simulink model "MMNNsExample1"  (R2014a)
settings: Solver=ode45  StartTime=0.0  StopTime=5  RelTol=1e-6
(part 2 of 2)

== system MMNNsExample1/b22(2)(x2(t))*f(x2(t-tau2(t)))/x2(t)*b22(x2(t)) ==
  In1 : Inport
  In2 : Inport  Port=2
  Product1 : Product  RndMeth=Zero
  Variable Time Delay : VariableTransportDelay  MaximumDelay=10  MaximumPoints=2^20
  f(x(t))=0.5*(|x+1|-|x-1|) : Subsystem
  tau2(t)=0.5+0.5*sin(t) : Subsystem
  Out1 : Outport
  wires:
  Product1/1 -> Out1/1
  f(x(t))=0.5*(|x+1|-|x-1|)/1(Out1) -> Variable Time Delay/1
  Variable Time Delay/1 -> Product1/2  "f2(x2(t-tau2(t)))"
  tau2(t)=0.5+0.5*sin(t)/1(Out1) -> Variable Time Delay/2
  In2/1 -> f(x(t))=0.5*(|x+1|-|x-1|)/1(In1)  "x2(t)"
  In1/1 -> Product1/1  "b22(x2(t))"

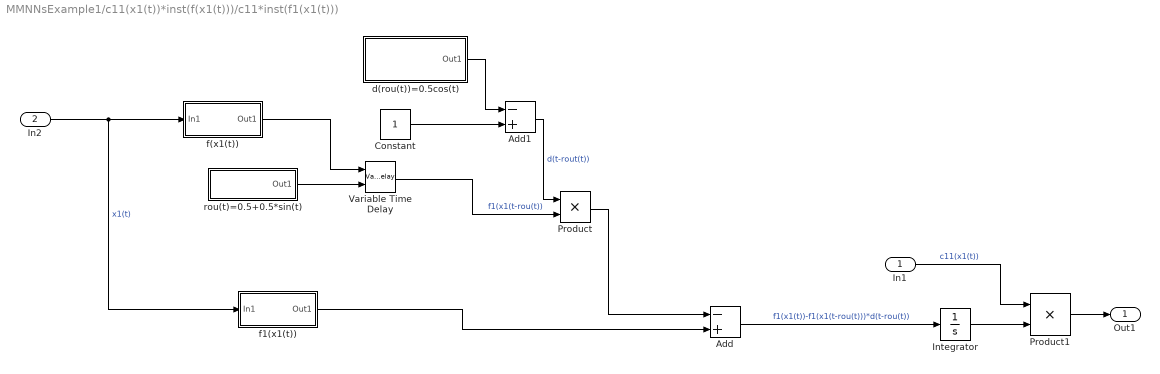
== system MMNNsExample1/c11(x1(t))*inst(f(x1(t)))/c11*inst(f1(x1(t))) ==
  In1 : Inport
  In2 : Inport  Port=2
  Add : Sum  Inputs=-+
  Add1 : Sum  Inputs=-+
  Constant : Constant
  Integrator : Integrator  InitialCondition=0.2
      settings: AttributesFormatString=|
      | %<Name>
      | %<InitialCondition>
  Product : Product
  Product1 : Product  RndMeth=Zero
  Variable Time Delay : VariableTransportDelay  MaximumDelay=10  MaximumPoints=2^21
  d(rou(t))=0.5cos(t) : Subsystem
  f(x1(t)) : Subsystem
  f1(x1(t)) : Subsystem
  rou(t)=0.5+0.5*sin(t) : Subsystem
  Out1 : Outport
  wires:
  Product1/1 -> Out1/1
  f(x1(t))/1(Out1) -> Variable Time Delay/1
  rou(t)=0.5+0.5*sin(t)/1(Out1) -> Variable Time Delay/2
  f1(x1(t))/1(Out1) -> Add/2
  Constant/1 -> Add1/2
  d(rou(t))=0.5cos(t)/1(Out1) -> Add1/1
  Add1/1 -> Product/1  "d(t-rout(t))"
  Variable Time Delay/1 -> Product/2  "f1(x1(t-rou(t))"
  Product/1 -> Add/1
  Add/1 -> Integrator/1  "f1(x1(t))-f1(x1(t-rou(t)))*d(t-rou(t))"
  Integrator/1 -> Product1/2
  In2/1 -> f1(x1(t))/1(In1), f(x1(t))/1(In1)  "x1(t)"
  In1/1 -> Product1/1  "c11(x1(t))"

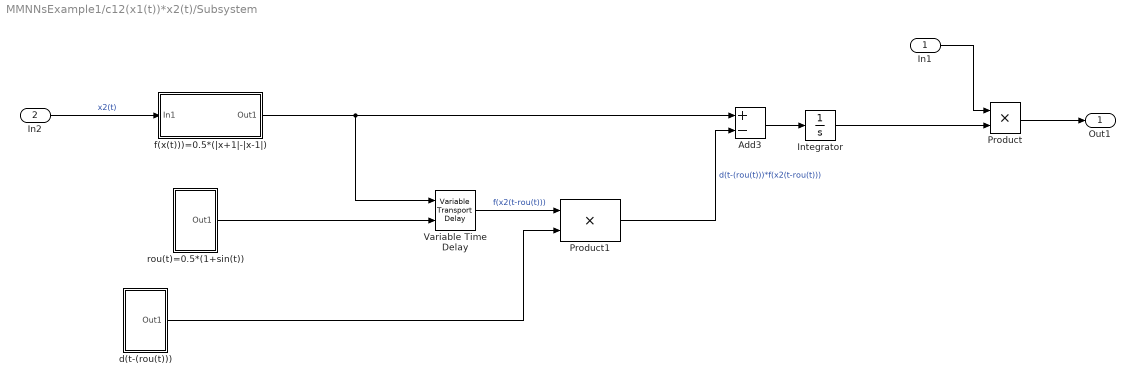
== system MMNNsExample1/c12(x1(t))*x2(t)/Subsystem ==
  In1 : Inport
      settings: AttributesFormatString=%<Name>
  In2 : Inport  Port=2
      settings: AttributesFormatString=%<Name>
  Add3 : Sum  Inputs=+-
  Integrator : Integrator  InitialCondition=0.3
      settings: AttributesFormatString=|
      | %<Name>
      | %<InitialCondition>
  Product : Product
  Product1 : Product
  Variable Time Delay : VariableTransportDelay  MaximumDelay=10  MaximumPoints=2^21
      settings: AttributesFormatString=%<Name>
  d(t-(rou(t))) : Subsystem
  f(x(t)))=0.5*(|x+1|-|x-1|) : Subsystem
  rou(t)=0.5*(1+sin(t)) : Subsystem
  Out1 : Outport
      settings: AttributesFormatString=%<Name>
  wires:
  f(x(t)))=0.5*(|x+1|-|x-1|)/1(Out1) -> Variable Time Delay/1, Add3/1
  Add3/1 -> Integrator/1
  d(t-(rou(t)))/1(Out1) -> Product1/2
  rou(t)=0.5*(1+sin(t))/1(Out1) -> Variable Time Delay/2
  Variable Time Delay/1 -> Product1/1  "f(x2(t-rou(t)))"
  Product1/1 -> Add3/2  "d(t-(rou(t)))*f(x2(t-rou(t)))"
  Integrator/1 -> Product/2
  In1/1 -> Product/1
  In2/1 -> f(x(t)))=0.5*(|x+1|-|x-1|)/1(In1)  "x2(t)"
  Product/1 -> Out1/1

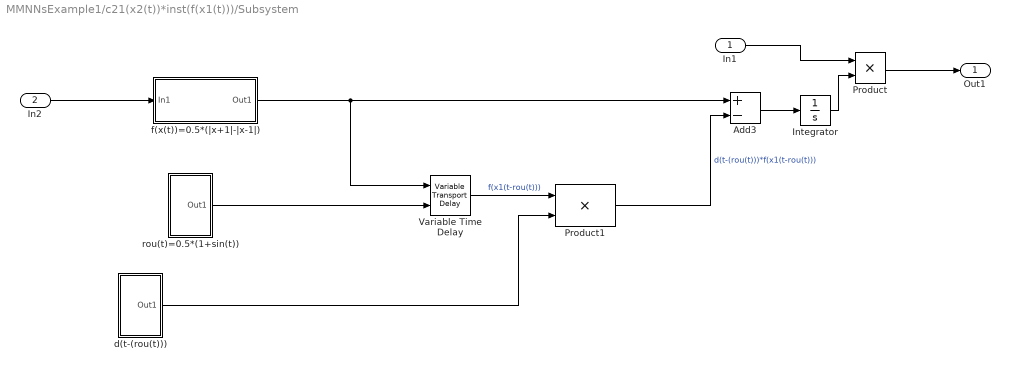
== system MMNNsExample1/c21(x2(t))*inst(f(x1(t)))/Subsystem ==
  In1 : Inport
  In2 : Inport  Port=2
  Add3 : Sum  Inputs=+-
  Integrator : Integrator  InitialCondition=0.2
      settings: AttributesFormatString=|
      | %<Name>
      | %<InitialCondition>
  Product : Product
  Product1 : Product
  Variable Time Delay : VariableTransportDelay  MaximumDelay=10  MaximumPoints=2^21
      settings: AttributesFormatString=%<Name>
  d(t-(rou(t))) : Subsystem
  f(x(t))=0.5*(|x+1|-|x-1|) : Subsystem
  rou(t)=0.5*(1+sin(t)) : Subsystem
  Out1 : Outport
  wires:
  Variable Time Delay/1 -> Product1/1  "f(x1(t-rou(t)))"
  f(x(t))=0.5*(|x+1|-|x-1|)/1(Out1) -> Variable Time Delay/1, Add3/1
  d(t-(rou(t)))/1(Out1) -> Product1/2
  Add3/1 -> Integrator/1
  rou(t)=0.5*(1+sin(t))/1(Out1) -> Variable Time Delay/2
  Product1/1 -> Add3/2  "d(t-(rou(t)))*f(x1(t-rou(t)))"
  Integrator/1 -> Product/2
  Product/1 -> Out1/1
  In1/1 -> Product/1
  In2/1 -> f(x(t))=0.5*(|x+1|-|x-1|)/1(In1)

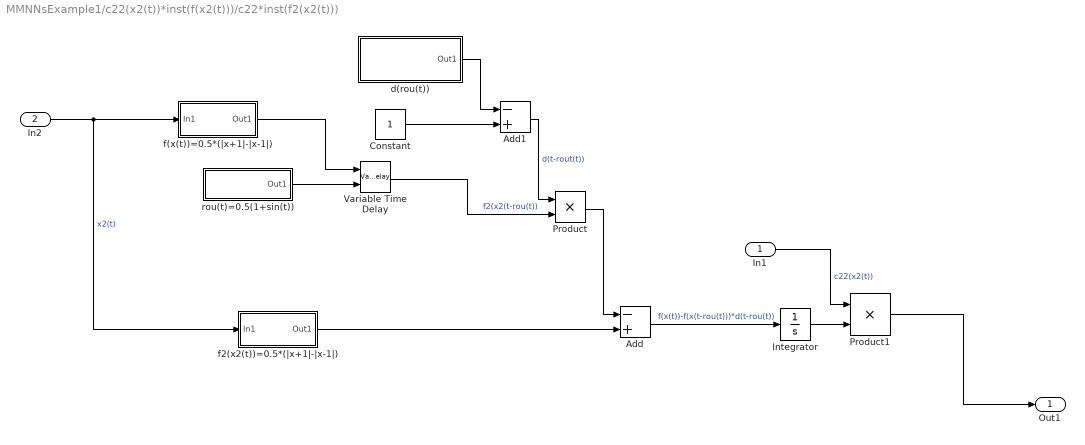
== system MMNNsExample1/c22(x2(t))*inst(f(x2(t)))/c22*inst(f2(x2(t))) ==
  In1 : Inport
  In2 : Inport  Port=2
  Add : Sum  Inputs=-+
  Add1 : Sum  Inputs=-+
  Constant : Constant
  Integrator : Integrator  InitialCondition=0.3
      settings: AttributesFormatString=|
      | %<Name>
      | %<InitialCondition>
  Product : Product
  Product1 : Product  RndMeth=Zero
  Variable Time Delay : VariableTransportDelay  MaximumDelay=10  MaximumPoints=2^21
  d(rou(t)) : Subsystem
  f(x(t))=0.5*(|x+1|-|x-1|) : Subsystem
  f2(x2(t))=0.5*(|x+1|-|x-1|) : Subsystem
  rou(t)=0.5(1+sin(t)) : Subsystem
  Out1 : Outport
  wires:
  Product1/1 -> Out1/1
  f(x(t))=0.5*(|x+1|-|x-1|)/1(Out1) -> Variable Time Delay/1
  rou(t)=0.5(1+sin(t))/1(Out1) -> Variable Time Delay/2
  f2(x2(t))=0.5*(|x+1|-|x-1|)/1(Out1) -> Add/2
  Constant/1 -> Add1/2
  d(rou(t))/1(Out1) -> Add1/1
  Add1/1 -> Product/1  "d(t-rout(t))"
  Variable Time Delay/1 -> Product/2  "f2(x2(t-rou(t))"
  Product/1 -> Add/1
  Add/1 -> Integrator/1  "f(x(t))-f(x(t-rou(t)))*d(t-rou(t))"
  Integrator/1 -> Product1/2
  In2/1 -> f2(x2(t))=0.5*(|x+1|-|x-1|)/1(In1), f(x(t))=0.5*(|x+1|-|x-1|)/1(In1)  "x2(t)"
  In1/1 -> Product1/1  "c22(x2(t))"

== system MMNNsExample1/22c21(y2(t))*inst(f(y1(t))/Subsystem/d(t-(rou(t))) ==
  Add : Sum  Inputs=+-
  Clock : Clock
  Constant2 : Constant
  Gain : Gain  Gain=0.5
  Sine Wave Function : Sin  TimeSource=Use external signal  Phase=0.5*pi  SampleTime=0
      settings: AttributesFormatString=%<Name>
  Out1 : Outport
  wires:
  Clock/1 -> Sine Wave Function/1
  Constant2/1 -> Add/1
  Gain/1 -> Add/2
  Add/1 -> Out1/1
  Sine Wave Function/1 -> Gain/1  "cos(t)"

== system MMNNsExample1/22c21(y2(t))*inst(f(y1(t))/Subsystem/f(x(t))=0.5*(|x+1|-|x-1|) ==
  In1 : Inport
      settings: AttributesFormatString=%<Name>
  Abs : Abs
      settings: AttributesFormatString=%<Name>
  Abs1 : Abs
  Add : Sum
  Add1 : Sum  Inputs=-+
  Add2 : Sum  Inputs=+-
  Constant : Constant
  Gain : Gain  Gain=0.5
  Out1 : Outport
      settings: AttributesFormatString=%<Name>
  wires:
  Gain/1 -> Out1/1
  Abs/1 -> Add2/1
  Add2/1 -> Gain/1
  Add1/1 -> Abs1/1
  In1/1 -> Add1/2, Add/1
  Abs1/1 -> Add2/2
  Constant/1 -> Add1/1, Add/2
  Add/1 -> Abs/1

== system MMNNsExample1/22c21(y2(t))*inst(f(y1(t))/Subsystem/rou(t)=0.5*(1+sin(t)) ==
  Add2 : Sum
  Clock1 : Clock
  Constant3 : Constant
  Gain1 : Gain  Gain=0.5
  Sine Wave Function1 : Sin  TimeSource=Use external signal  SampleTime=0
      settings: AttributesFormatString=%<Name>
  Out1 : Outport
  wires:
  Constant3/1 -> Add2/2
  Sine Wave Function1/1 -> Add2/1  "sin(t)"
  Gain1/1 -> Out1/1
  Add2/1 -> Gain1/1
  Clock1/1 -> Sine Wave Function1/1

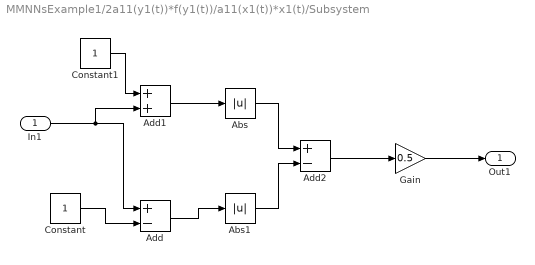
== system MMNNsExample1/2a11(y1(t))*f(y1(t))/a11(x1(t))*x1(t)/Subsystem ==
  In1 : Inport
  Abs : Abs
  Abs1 : Abs
  Add : Sum  Inputs=+-
  Add1 : Sum
  Add2 : Sum  Inputs=+-
  Constant : Constant
  Constant1 : Constant
  Gain : Gain  Gain=0.5
  Out1 : Outport
  wires:
  Constant1/1 -> Add1/1
  In1/1 -> Add/1, Add1/2
  Add1/1 -> Abs/1
  Abs/1 -> Add2/1
  Constant/1 -> Add/2
  Add/1 -> Abs1/1
  Abs1/1 -> Add2/2
  Add2/1 -> Gain/1
  Gain/1 -> Out1/1

== system MMNNsExample1/2a12(y1(t))*f(y2(t))/Subsystem/f(x2(t)) ==
  In1 : Inport
  Abs : Abs
  Abs1 : Abs
  Add : Sum
  Add1 : Sum  Inputs=-+
  Add2 : Sum  Inputs=+-
  Constant : Constant
  Gain : Gain  Gain=0.5
  Out1 : Outport
  wires:
  In1/1 -> Add1/2, Add/1  "x2(t)"
  Constant/1 -> Add1/1, Add/2
  Add/1 -> Abs/1
  Add1/1 -> Abs1/1
  Abs/1 -> Add2/1
  Abs1/1 -> Add2/2
  Add2/1 -> Gain/1  "f=(|x+1|-|x-1|)/2"
  Gain/1 -> Out1/1

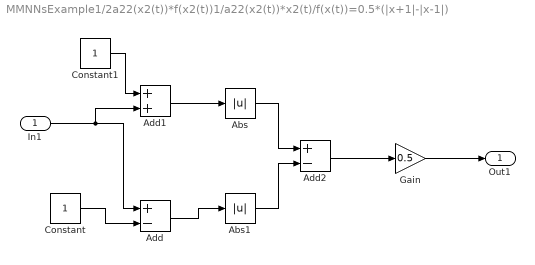
== system MMNNsExample1/2a22(x2(t))*f(x2(t))1/a22(x2(t))*x2(t)/f(x(t))=0.5*(|x+1|-|x-1|) ==
  In1 : Inport
  Abs : Abs
  Abs1 : Abs
  Add : Sum  Inputs=+-
  Add1 : Sum
  Add2 : Sum  Inputs=+-
  Constant : Constant
  Constant1 : Constant
  Gain : Gain  Gain=0.5
  Out1 : Outport
  wires:
  Constant1/1 -> Add1/1
  In1/1 -> Add/1, Add1/2
  Add1/1 -> Abs/1
  Abs/1 -> Add2/1
  Constant/1 -> Add/2
  Add/1 -> Abs1/1
  Abs1/1 -> Add2/2
  Add2/1 -> Gain/1
  Gain/1 -> Out1/1

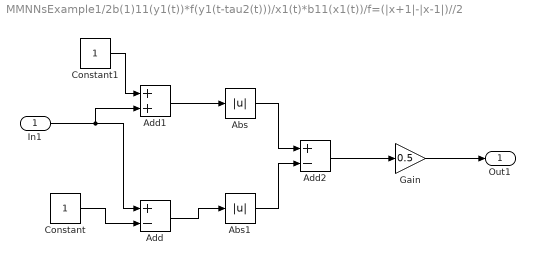
== system MMNNsExample1/2b(1)11(y1(t))*f(y1(t-tau2(t)))/x1(t)*b11(x1(t))/f=(|x+1|-|x-1|)//2 ==
  In1 : Inport
  Abs : Abs
  Abs1 : Abs
  Add : Sum  Inputs=+-
  Add1 : Sum
  Add2 : Sum  Inputs=+-
  Constant : Constant
  Constant1 : Constant
  Gain : Gain  Gain=0.5
  Out1 : Outport
  wires:
  Constant1/1 -> Add1/1
  In1/1 -> Add/1, Add1/2
  Add1/1 -> Abs/1
  Abs/1 -> Add2/1
  Constant/1 -> Add/2
  Add/1 -> Abs1/1
  Abs1/1 -> Add2/2
  Add2/1 -> Gain/1
  Gain/1 -> Out1/1

== system MMNNsExample1/2b(1)11(y1(t))*f(y1(t-tau2(t)))/x1(t)*b11(x1(t))/tau2(t)=0.5+0.5*sin(t) ==
  Add : Sum
  Clock : Clock
  Constant : Constant
  Gain : Gain
  Gain1 : Gain  Gain=0.5
  Sine Wave Function : Sin  TimeSource=Use external signal  SampleTime=0
      settings: AttributesFormatString=%<Name>
  tau(t)=0.5+0.5*sin(t) : Outport
  wires:
  Sine Wave Function/1 -> Gain/1  "sin(t)"
  Constant/1 -> Add/2
  Clock/1 -> Sine Wave Function/1
  Add/1 -> Gain1/1
  Gain/1 -> Add/1
  Gain1/1 -> tau(t)=0.5+0.5*sin(t)/1

== system MMNNsExample1/2b(1)21(y2(t))*f(y1(t-tau1(t)))1/Subsystem/f(x(t))=0.5*(|x+1|-|x-1|) ==
  In1 : Inport
      settings: AttributesFormatString=%<Name>
  Abs : Abs
      settings: AttributesFormatString=%<Name>
  Abs1 : Abs
  Add : Sum
  Add1 : Sum  Inputs=-+
  Add2 : Sum  Inputs=+-
  Constant : Constant
  Gain : Gain  Gain=0.5
  Out1 : Outport
      settings: AttributesFormatString=%<Name>
  wires:
  Gain/1 -> Out1/1
  Abs/1 -> Add2/1
  Add2/1 -> Gain/1
  Add1/1 -> Abs1/1
  In1/1 -> Add1/2, Add/1
  Abs1/1 -> Add2/2
  Constant/1 -> Add1/1, Add/2
  Add/1 -> Abs/1

== system MMNNsExample1/2b(1)21(y2(t))*f(y1(t-tau1(t)))1/Subsystem/tau(t)=0.5+0.5*cos(t) ==
  Add : Sum
  Clock : Clock
  Constant2 : Constant
  Gain : Gain  Gain=0.5
  Sine Wave Function : Sin  TimeSource=Use external signal  Phase=0.5*pi  SampleTime=0
      settings: AttributesFormatString=%<Name>
  Out1 : Outport
  wires:
  Clock/1 -> Sine Wave Function/1
  Gain/1 -> Out1/1
  Constant2/1 -> Add/1
  Add/1 -> Gain/1
  Sine Wave Function/1 -> Add/2  "cos(t)"

== system MMNNsExample1/2b(1)22(y2(t))*f(y2(t-tau(t))1/x2(t)*b22(x2(t))/f(x(t))=0.5*(|x+1|-|x-1|) ==
  In1 : Inport
  Abs : Abs
  Abs1 : Abs
  Add : Sum  Inputs=+-
  Add1 : Sum
  Add2 : Sum  Inputs=+-
  Constant : Constant
  Constant1 : Constant
  Gain : Gain  Gain=0.5
  Out1 : Outport
  wires:
  Constant1/1 -> Add1/1
  In1/1 -> Add/1, Add1/2
  Add1/1 -> Abs/1
  Abs/1 -> Add2/1
  Constant/1 -> Add/2
  Add/1 -> Abs1/1
  Abs1/1 -> Add2/2
  Add2/1 -> Gain/1
  Gain/1 -> Out1/1

== system MMNNsExample1/2b(1)22(y2(t))*f(y2(t-tau(t))1/x2(t)*b22(x2(t))/tau(t)=0.5+0.5*cos(t) ==
  Add : Sum
  Clock : Clock
  Constant : Constant
  Gain : Gain
  Gain1 : Gain  Gain=0.5
  Sine Wave Function : Sin  TimeSource=Use external signal  Phase=0.5*pi  SampleTime=0
      settings: AttributesFormatString=%<Name>
  Out1 : Outport
  wires:
  Add/1 -> Gain1/1
  Clock/1 -> Sine Wave Function/1
  Sine Wave Function/1 -> Gain/1  "cos(t)"
  Constant/1 -> Add/2
  Gain/1 -> Add/1
  Gain1/1 -> Out1/1  "tau(t)=0.5+0.5*cos(t)"

== system MMNNsExample1/2b(2)12(y1(t))*f(y2(t-tau2(t)))/Subsystem/f=(|x+1|-|x-1|)//2 ==
  In1 : Inport
      settings: AttributesFormatString=%<Name>
  Abs : Abs
      settings: AttributesFormatString=%<Name>
  Abs1 : Abs
  Add : Sum
  Add1 : Sum  Inputs=-+
  Add2 : Sum  Inputs=+-
  Constant : Constant
  Gain : Gain  Gain=0.5
  Out1 : Outport
      settings: AttributesFormatString=%<Name>
  wires:
  Gain/1 -> Out1/1
  Abs/1 -> Add2/1
  Add2/1 -> Gain/1
  Add1/1 -> Abs1/1
  In1/1 -> Add1/2, Add/1
  Abs1/1 -> Add2/2
  Constant/1 -> Add1/1, Add/2
  Add/1 -> Abs/1

== system MMNNsExample1/2b(2)12(y1(t))*f(y2(t-tau2(t)))/Subsystem/tau(t)=0.5+0.5*sin(t) ==
  Add : Sum
  Clock : Clock
  Constant2 : Constant
  Gain : Gain  Gain=0.5
  Sine Wave Function : Sin  TimeSource=Use external signal  SampleTime=0
      settings: AttributesFormatString=%<Name>
  Out1 : Outport
  wires:
  Clock/1 -> Sine Wave Function/1
  Gain/1 -> Out1/1  "tau(t)=0.5+0.5*sin(t)"
  Constant2/1 -> Add/1
  Add/1 -> Gain/1
  Sine Wave Function/1 -> Add/2  "sin(t)"

== system MMNNsExample1/2b(2)21(y2(t))*f(y1(t-tau2(t)))1/Subsystem/f(x(t))=0.5*(|x+1|-|x-1|) ==
  In1 : Inport
      settings: AttributesFormatString=%<Name>
  Abs : Abs
      settings: AttributesFormatString=%<Name>
  Abs1 : Abs
  Add : Sum
  Add1 : Sum  Inputs=-+
  Add2 : Sum  Inputs=+-
  Constant : Constant
  Gain : Gain  Gain=0.5
  Out1 : Outport
      settings: AttributesFormatString=%<Name>
  wires:
  Gain/1 -> Out1/1
  Abs/1 -> Add2/1
  Add2/1 -> Gain/1
  Add1/1 -> Abs1/1
  In1/1 -> Add1/2, Add/1
  Abs1/1 -> Add2/2
  Constant/1 -> Add1/1, Add/2
  Add/1 -> Abs/1

== system MMNNsExample1/2b(2)21(y2(t))*f(y1(t-tau2(t)))1/Subsystem/tau(t)=0.5+0.5*sin(t) ==
  Add : Sum
  Clock : Clock
  Constant2 : Constant
  Gain : Gain  Gain=0.5
  Sine Wave Function : Sin  TimeSource=Use external signal  SampleTime=0
      settings: AttributesFormatString=%<Name>
  Out1 : Outport
  wires:
  Clock/1 -> Sine Wave Function/1
  Gain/1 -> Out1/1
  Constant2/1 -> Add/1
  Add/1 -> Gain/1
  Sine Wave Function/1 -> Add/2  "sin(t)"

== system MMNNsExample1/2b(2)22(y2(t))*f(y2(t-tau2(t))/x2(t)*b22(x2(t))/f(x(t))=0.5*(|x+1|-|x-1|) ==
  In1 : Inport
  Abs : Abs
  Abs1 : Abs
  Add : Sum  Inputs=+-
  Add1 : Sum
  Add2 : Sum  Inputs=+-
  Constant : Constant
  Constant1 : Constant
  Gain : Gain  Gain=0.5
  Out1 : Outport
  wires:
  Constant1/1 -> Add1/1
  In1/1 -> Add/1, Add1/2
  Add1/1 -> Abs/1
  Abs/1 -> Add2/1
  Constant/1 -> Add/2
  Add/1 -> Abs1/1
  Abs1/1 -> Add2/2
  Add2/1 -> Gain/1
  Gain/1 -> Out1/1

== system MMNNsExample1/2b(2)22(y2(t))*f(y2(t-tau2(t))/x2(t)*b22(x2(t))/tau(t)=0.5+0.5*sin(t) ==
  Add : Sum
  Clock : Clock
  Constant : Constant
  Gain : Gain
  Gain1 : Gain  Gain=0.5
  Sine Wave Function : Sin  TimeSource=Use external signal  SampleTime=0
      settings: AttributesFormatString=%<Name>
  Out1 : Outport
  wires:
  Add/1 -> Gain1/1
  Clock/1 -> Sine Wave Function/1
  Sine Wave Function/1 -> Gain/1  "sin(t)"
  Constant/1 -> Add/2
  Gain/1 -> Add/1
  Gain1/1 -> Out1/1  "tau(t)=0.5+0.5*sin(t)"

== system MMNNsExample1/2b11(y1(t))*f(y1(t-tau(t)))/x1(t)*b11(x1(t))/f=(|x+1|-|x-1|)//2 ==
  In1 : Inport
  Abs : Abs
  Abs1 : Abs
  Add : Sum  Inputs=+-
  Add1 : Sum
  Add2 : Sum  Inputs=+-
  Constant : Constant
  Constant1 : Constant
  Gain : Gain  Gain=0.5
  Out1 : Outport
  wires:
  Constant1/1 -> Add1/1
  In1/1 -> Add/1, Add1/2
  Add1/1 -> Abs/1
  Abs/1 -> Add2/1
  Constant/1 -> Add/2
  Add/1 -> Abs1/1
  Abs1/1 -> Add2/2
  Add2/1 -> Gain/1
  Gain/1 -> Out1/1

== system MMNNsExample1/2b11(y1(t))*f(y1(t-tau(t)))/x1(t)*b11(x1(t))/tau(t)=0.5+0.5*cos(t) ==
  Add : Sum
  Clock : Clock
  Constant : Constant
  Gain : Gain
  Gain1 : Gain  Gain=0.5
  Sine Wave Function : Sin  TimeSource=Use external signal  Phase=0.5*pi  SampleTime=0
      settings: AttributesFormatString=%<Name>
  tau(t)=0.5+0.5*cos(t) : Outport
  wires:
  Sine Wave Function/1 -> Gain/1  "cos(t)"
  Constant/1 -> Add/2
  Clock/1 -> Sine Wave Function/1
  Add/1 -> Gain1/1
  Gain/1 -> Add/1
  Gain1/1 -> tau(t)=0.5+0.5*cos(t)/1

== system MMNNsExample1/2b12(y1(t))*f(y2(t-tau1(t)))/Subsystem/f=(|x+1|-|x-1|)//2 ==
  In1 : Inport
      settings: AttributesFormatString=%<Name>
  Abs : Abs
      settings: AttributesFormatString=%<Name>
  Abs1 : Abs
  Add : Sum
  Add1 : Sum  Inputs=-+
  Add2 : Sum  Inputs=+-
  Constant : Constant
  Gain : Gain  Gain=0.5
  Out1 : Outport
      settings: AttributesFormatString=%<Name>
  wires:
  Gain/1 -> Out1/1
  Abs/1 -> Add2/1
  Add2/1 -> Gain/1
  Add1/1 -> Abs1/1
  In1/1 -> Add1/2, Add/1
  Abs1/1 -> Add2/2
  Constant/1 -> Add1/1, Add/2
  Add/1 -> Abs/1

== system MMNNsExample1/2b12(y1(t))*f(y2(t-tau1(t)))/Subsystem/tau(t)=0.5+0.5*cos(t) ==
  Add : Sum
  Clock : Clock
  Constant2 : Constant
  Gain : Gain  Gain=0.5
  Sine Wave Function : Sin  TimeSource=Use external signal  Phase=0.5*pi  SampleTime=0
      settings: AttributesFormatString=%<Name>
  Out1 : Outport
  wires:
  Clock/1 -> Sine Wave Function/1
  Gain/1 -> Out1/1  "tau(t)=0.5+0.5*cos(t)"
  Constant2/1 -> Add/1
  Add/1 -> Gain/1
  Sine Wave Function/1 -> Add/2  "cos(t)"

== system MMNNsExample1/2c11(y1(t))*inst(f(y1(t)))1/c11*inst(f1(x1(t)))/d(rou(t))=0.5cos(t) ==
  Clock : Clock
  Gain : Gain  Gain=0.5
  Sine Wave Function : Sin  TimeSource=Use external signal  Phase=0.5*pi  SampleTime=0
  Out1 : Outport
  wires:
  Sine Wave Function/1 -> Gain/1  "cos(t)"
  Gain/1 -> Out1/1  "rou(t)=d(0.5+0.5*sin(t))"
  Clock/1 -> Sine Wave Function/1

== system MMNNsExample1/2c11(y1(t))*inst(f(y1(t)))1/c11*inst(f1(x1(t)))/f(x1(t)) ==
  In1 : Inport
  Abs : Abs
  Abs1 : Abs
  Add : Sum  Inputs=+-
  Add1 : Sum
  Add2 : Sum  Inputs=+-
  Constant1 : Constant
  Gain : Gain  Gain=0.5
  Out1 : Outport
  wires:
  Constant1/1 -> Add/2, Add1/1
  In1/1 -> Add/1, Add1/2  "x1(t)"
  Add1/1 -> Abs/1
  Abs/1 -> Add2/1
  Add/1 -> Abs1/1
  Abs1/1 -> Add2/2
  Add2/1 -> Gain/1
  Gain/1 -> Out1/1

== system MMNNsExample1/2c11(y1(t))*inst(f(y1(t)))1/c11*inst(f1(x1(t)))/f1(x1(t)) ==
  In1 : Inport
  Abs : Abs
  Abs1 : Abs
  Add : Sum  Inputs=+-
  Add1 : Sum
  Add2 : Sum  Inputs=+-
  Constant : Constant
  Constant1 : Constant
  Gain : Gain  Gain=0.5
  Out1 : Outport
  wires:
  Gain/1 -> Out1/1
  Add2/1 -> Gain/1
  Abs1/1 -> Add2/2
  Add/1 -> Abs1/1
  Constant/1 -> Add/2
  Abs/1 -> Add2/1
  Add1/1 -> Abs/1
  In1/1 -> Add1/2, Add/1
  Constant1/1 -> Add1/1

== system MMNNsExample1/2c11(y1(t))*inst(f(y1(t)))1/c11*inst(f1(x1(t)))/rou(t)=0.5+0.5*sin(t) ==
  Add : Sum
  Clock : Clock
  Constant : Constant
  Gain : Gain
  Gain1 : Gain  Gain=0.5
  Sine Wave Function : Sin  TimeSource=Use external signal  SampleTime=0
  Out1 : Outport
  wires:
  Clock/1 -> Sine Wave Function/1
  Constant/1 -> Add/2
  Gain/1 -> Add/1
  Add/1 -> Gain1/1
  Sine Wave Function/1 -> Gain/1  "sin(t)"
  Gain1/1 -> Out1/1

== system MMNNsExample1/2c12(y1(t))*inst(f(y2(t))))1/Subsystem/d(t-(rou(t))) ==
  Add : Sum  Inputs=+-
  Clock : Clock
  Constant2 : Constant
  Gain : Gain  Gain=0.5
  Sine Wave Function : Sin  TimeSource=Use external signal  Phase=0.5*pi  SampleTime=0
      settings: AttributesFormatString=%<Name>
  Out1 : Outport
  wires:
  Clock/1 -> Sine Wave Function/1
  Constant2/1 -> Add/1
  Gain/1 -> Add/2
  Add/1 -> Out1/1
  Sine Wave Function/1 -> Gain/1  "cos(t)"

== system MMNNsExample1/2c12(y1(t))*inst(f(y2(t))))1/Subsystem/f(x(t)))=0.5*(|x+1|-|x-1|) ==
  In1 : Inport
      settings: AttributesFormatString=%<Name>
  Abs : Abs
      settings: AttributesFormatString=%<Name>
  Abs1 : Abs
  Add : Sum
  Add1 : Sum  Inputs=-+
  Add2 : Sum  Inputs=+-
  Constant : Constant
  Gain : Gain  Gain=0.5
  Out1 : Outport
      settings: AttributesFormatString=%<Name>
  wires:
  Gain/1 -> Out1/1
  Abs/1 -> Add2/1
  Add2/1 -> Gain/1
  Add1/1 -> Abs1/1
  In1/1 -> Add1/2, Add/1
  Abs1/1 -> Add2/2
  Constant/1 -> Add1/1, Add/2
  Add/1 -> Abs/1

== system MMNNsExample1/2c12(y1(t))*inst(f(y2(t))))1/Subsystem/rou(t)=0.5*(1+sin(t)) ==
  Add2 : Sum
  Clock1 : Clock
  Constant3 : Constant
  Gain1 : Gain  Gain=0.5
  Sine Wave Function1 : Sin  TimeSource=Use external signal  SampleTime=0
      settings: AttributesFormatString=%<Name>
  Out1 : Outport
  wires:
  Constant3/1 -> Add2/2
  Sine Wave Function1/1 -> Add2/1  "sin(t)"
  Gain1/1 -> Out1/1  "rou(t)=0.5*(1+sin(t))"
  Add2/1 -> Gain1/1
  Clock1/1 -> Sine Wave Function1/1

== system MMNNsExample1/2c22(y2(t))*inst(f(y2(t)))/c22*inst(f2(x2(t)))/d(rou(t)) ==
  Clock : Clock
  Gain : Gain  Gain=0.5
  Sine Wave Function : Sin  TimeSource=Use external signal  Phase=0.5*pi  SampleTime=0
  Out1 : Outport
  wires:
  Sine Wave Function/1 -> Gain/1  "cos(t)"
  Gain/1 -> Out1/1  "d(rou(t))=0.5*cos(t)"
  Clock/1 -> Sine Wave Function/1

== system MMNNsExample1/2c22(y2(t))*inst(f(y2(t)))/c22*inst(f2(x2(t)))/f(x(t))=0.5*(|x+1|-|x-1|) ==
  In1 : Inport
  Abs : Abs
  Abs1 : Abs
  Add : Sum  Inputs=+-
  Add1 : Sum
  Add2 : Sum  Inputs=+-
  Constant1 : Constant
  Gain : Gain  Gain=0.5
  Out1 : Outport
  wires:
  Constant1/1 -> Add/2, Add1/1
  In1/1 -> Add/1, Add1/2  "x1(t)"
  Add1/1 -> Abs/1
  Abs/1 -> Add2/1
  Add/1 -> Abs1/1
  Abs1/1 -> Add2/2
  Add2/1 -> Gain/1
  Gain/1 -> Out1/1

== system MMNNsExample1/2c22(y2(t))*inst(f(y2(t)))/c22*inst(f2(x2(t)))/f2(x2(t))=0.5*(|x+1|-|x-1|) ==
  In1 : Inport
  Abs : Abs
  Abs1 : Abs
  Add : Sum  Inputs=+-
  Add1 : Sum
  Add2 : Sum  Inputs=+-
  Constant : Constant
  Constant1 : Constant
  Gain : Gain  Gain=0.5
  Out1 : Outport
  wires:
  Gain/1 -> Out1/1
  Add2/1 -> Gain/1
  Abs1/1 -> Add2/2
  Add/1 -> Abs1/1
  Constant/1 -> Add/2
  Abs/1 -> Add2/1
  Add1/1 -> Abs/1
  In1/1 -> Add1/2, Add/1
  Constant1/1 -> Add1/1

== system MMNNsExample1/2c22(y2(t))*inst(f(y2(t)))/c22*inst(f2(x2(t)))/rou(t)=0.5(1+sin(t)) ==
  Add : Sum
  Clock : Clock
  Constant : Constant
  Gain : Gain  Gain=0.5
  Sine Wave Function : Sin  TimeSource=Use external signal  SampleTime=0
  Out1 : Outport
  wires:
  Clock/1 -> Sine Wave Function/1
  Constant/1 -> Add/2
  Add/1 -> Gain/1
  Sine Wave Function/1 -> Add/1  "sin(t)"
  Gain/1 -> Out1/1

== system MMNNsExample1/a11(x1(t))*f(x1(t))/a11(x1(t))*x1(t)/Subsystem ==
  In1 : Inport
  Abs : Abs
  Abs1 : Abs
  Add : Sum  Inputs=+-
  Add1 : Sum
  Add2 : Sum  Inputs=+-
  Constant : Constant
  Constant1 : Constant
  Gain : Gain  Gain=0.5
  Out1 : Outport
  wires:
  Constant1/1 -> Add1/1
  In1/1 -> Add/1, Add1/2
  Add1/1 -> Abs/1
  Abs/1 -> Add2/1
  Constant/1 -> Add/2
  Add/1 -> Abs1/1
  Abs1/1 -> Add2/2
  Add2/1 -> Gain/1
  Gain/1 -> Out1/1

== system MMNNsExample1/a12(x1(t))*f(x2(t))/Subsystem/f(x2(t)) ==
  In1 : Inport
  Abs : Abs
  Abs1 : Abs
  Add : Sum
  Add1 : Sum  Inputs=-+
  Add2 : Sum  Inputs=+-
  Constant : Constant
  Gain : Gain  Gain=0.5
  Out1 : Outport
  wires:
  In1/1 -> Add1/2, Add/1  "x2(t)"
  Constant/1 -> Add1/1, Add/2
  Add/1 -> Abs/1
  Add1/1 -> Abs1/1
  Abs/1 -> Add2/1
  Abs1/1 -> Add2/2
  Add2/1 -> Gain/1  "f=(|x+1|-|x-1|)/2"
  Gain/1 -> Out1/1

== system MMNNsExample1/a22(x2(t))*f(x2(t))/a22(x2(t))*x2(t)/f(x(t))=0.5*(|x+1|-|x-1|) ==
  In1 : Inport
  Abs : Abs
  Abs1 : Abs
  Add : Sum  Inputs=+-
  Add1 : Sum
  Add2 : Sum  Inputs=+-
  Constant : Constant
  Constant1 : Constant
  Gain : Gain  Gain=0.5
  Out1 : Outport
  wires:
  Constant1/1 -> Add1/1
  In1/1 -> Add/1, Add1/2
  Add1/1 -> Abs/1
  Abs/1 -> Add2/1
  Constant/1 -> Add/2
  Add/1 -> Abs1/1
  Abs1/1 -> Add2/2
  Add2/1 -> Gain/1
  Gain/1 -> Out1/1

== system MMNNsExample1/b(1)12(x1(t))*f(x2(t-tau1(t)))/Subsystem/f=(|x+1|-|x-1|)//2 ==
  In1 : Inport
      settings: AttributesFormatString=%<Name>
  Abs : Abs
      settings: AttributesFormatString=%<Name>
  Abs1 : Abs
  Add : Sum
  Add1 : Sum  Inputs=-+
  Add2 : Sum  Inputs=+-
  Constant : Constant
  Gain : Gain  Gain=0.5
  Out1 : Outport
      settings: AttributesFormatString=%<Name>
  wires:
  Gain/1 -> Out1/1
  Abs/1 -> Add2/1
  Add2/1 -> Gain/1
  Add1/1 -> Abs1/1
  In1/1 -> Add1/2, Add/1
  Abs1/1 -> Add2/2
  Constant/1 -> Add1/1, Add/2
  Add/1 -> Abs/1

== system MMNNsExample1/b(1)12(x1(t))*f(x2(t-tau1(t)))/Subsystem/tau(t)=0.5+0.5*cos(t) ==
  Add : Sum
  Clock : Clock
  Constant2 : Constant
  Gain : Gain  Gain=0.5
  Sine Wave Function : Sin  TimeSource=Use external signal  Phase=0.5*pi  SampleTime=0
      settings: AttributesFormatString=%<Name>
  Out1 : Outport
  wires:
  Clock/1 -> Sine Wave Function/1
  Gain/1 -> Out1/1  "tau(t)=0.5+0.5*cos(t)"
  Constant2/1 -> Add/1
  Add/1 -> Gain/1
  Sine Wave Function/1 -> Add/2  "cos(t)"

== system MMNNsExample1/b(1)21(x2(t))*f(x1(t-tau1(t)))/Subsystem/f(x(t))=0.5*(|x+1|-|x-1|) ==
  In1 : Inport
      settings: AttributesFormatString=%<Name>
  Abs : Abs
      settings: AttributesFormatString=%<Name>
  Abs1 : Abs
  Add : Sum
  Add1 : Sum  Inputs=-+
  Add2 : Sum  Inputs=+-
  Constant : Constant
  Gain : Gain  Gain=0.5
  Out1 : Outport
      settings: AttributesFormatString=%<Name>
  wires:
  Gain/1 -> Out1/1
  Abs/1 -> Add2/1
  Add2/1 -> Gain/1
  Add1/1 -> Abs1/1
  In1/1 -> Add1/2, Add/1
  Abs1/1 -> Add2/2
  Constant/1 -> Add1/1, Add/2
  Add/1 -> Abs/1

== system MMNNsExample1/b(1)21(x2(t))*f(x1(t-tau1(t)))/Subsystem/tau(t)=0.5+0.5*cos(t) ==
  Add : Sum
  Clock : Clock
  Constant2 : Constant
  Gain : Gain  Gain=0.5
  Sine Wave Function : Sin  TimeSource=Use external signal  Phase=0.5*pi  SampleTime=0
      settings: AttributesFormatString=%<Name>
  Out1 : Outport
  wires:
  Clock/1 -> Sine Wave Function/1
  Gain/1 -> Out1/1
  Constant2/1 -> Add/1
  Add/1 -> Gain/1
  Sine Wave Function/1 -> Add/2  "cos(t)"

== system MMNNsExample1/b(2)11(x1(t))*f(x1(t-tau2t)))/x1(t)*b11(x1(t))/f=(|x+1|-|x-1|)//2 ==
  In1 : Inport
  Abs : Abs
  Abs1 : Abs
  Add : Sum  Inputs=+-
  Add1 : Sum
  Add2 : Sum  Inputs=+-
  Constant : Constant
  Constant1 : Constant
  Gain : Gain  Gain=0.5
  Out1 : Outport
  wires:
  Constant1/1 -> Add1/1
  In1/1 -> Add/1, Add1/2
  Add1/1 -> Abs/1
  Abs/1 -> Add2/1
  Constant/1 -> Add/2
  Add/1 -> Abs1/1
  Abs1/1 -> Add2/2
  Add2/1 -> Gain/1
  Gain/1 -> Out1/1

== system MMNNsExample1/b(2)11(x1(t))*f(x1(t-tau2t)))/x1(t)*b11(x1(t))/tau2(t)=0.5+0.5*sin(t) ==
  Add : Sum
  Clock : Clock
  Constant : Constant
  Gain : Gain
  Gain1 : Gain  Gain=0.5
  Sine Wave Function : Sin  TimeSource=Use external signal  SampleTime=0
      settings: AttributesFormatString=%<Name>
  tau(t)=0.5+0.5*sin(t) : Outport
  wires:
  Sine Wave Function/1 -> Gain/1  "sin(t)"
  Constant/1 -> Add/2
  Clock/1 -> Sine Wave Function/1
  Add/1 -> Gain1/1
  Gain/1 -> Add/1
  Gain1/1 -> tau(t)=0.5+0.5*sin(t)/1

== system MMNNsExample1/b(2)12(x1(t))*f(x2(t-tau2(t)))/Subsystem/f=(|x+1|-|x-1|)//2 ==
  In1 : Inport
      settings: AttributesFormatString=%<Name>
  Abs : Abs
      settings: AttributesFormatString=%<Name>
  Abs1 : Abs
  Add : Sum
  Add1 : Sum  Inputs=-+
  Add2 : Sum  Inputs=+-
  Constant : Constant
  Gain : Gain  Gain=0.5
  Out1 : Outport
      settings: AttributesFormatString=%<Name>
  wires:
  Gain/1 -> Out1/1
  Abs/1 -> Add2/1
  Add2/1 -> Gain/1
  Add1/1 -> Abs1/1
  In1/1 -> Add1/2, Add/1
  Abs1/1 -> Add2/2
  Constant/1 -> Add1/1, Add/2
  Add/1 -> Abs/1

== system MMNNsExample1/b(2)12(x1(t))*f(x2(t-tau2(t)))/Subsystem/tau2(t)=0.5+0.5*sin(t) ==
  Add : Sum
  Clock : Clock
  Constant2 : Constant
  Gain : Gain  Gain=0.5
  Sine Wave Function : Sin  TimeSource=Use external signal  SampleTime=0
      settings: AttributesFormatString=%<Name>
  Out1 : Outport
  wires:
  Clock/1 -> Sine Wave Function/1
  Gain/1 -> Out1/1  "tau2(t)=0.5+0.5*sin(t)"
  Constant2/1 -> Add/1
  Add/1 -> Gain/1
  Sine Wave Function/1 -> Add/2  "sin(t)"

== system MMNNsExample1/b(2)21(x2(t))*f(x1(t-tau2(t)))/Subsystem/f(x(t))=0.5*(|x+1|-|x-1|) ==
  In1 : Inport
      settings: AttributesFormatString=%<Name>
  Abs : Abs
      settings: AttributesFormatString=%<Name>
  Abs1 : Abs
  Add : Sum
  Add1 : Sum  Inputs=-+
  Add2 : Sum  Inputs=+-
  Constant : Constant
  Gain : Gain  Gain=0.5
  Out1 : Outport
      settings: AttributesFormatString=%<Name>
  wires:
  Gain/1 -> Out1/1
  Abs/1 -> Add2/1
  Add2/1 -> Gain/1
  Add1/1 -> Abs1/1
  In1/1 -> Add1/2, Add/1
  Abs1/1 -> Add2/2
  Constant/1 -> Add1/1, Add/2
  Add/1 -> Abs/1

== system MMNNsExample1/b(2)21(x2(t))*f(x1(t-tau2(t)))/Subsystem/tau2(t)=0.5+0.5*sin(t) ==
  Add : Sum
  Clock : Clock
  Constant2 : Constant
  Gain : Gain  Gain=0.5
  Sine Wave Function : Sin  TimeSource=Use external signal  SampleTime=0
      settings: AttributesFormatString=%<Name>
  Out1 : Outport
  wires:
  Clock/1 -> Sine Wave Function/1
  Gain/1 -> Out1/1
  Constant2/1 -> Add/1
  Add/1 -> Gain/1
  Sine Wave Function/1 -> Add/2  "sin(t)"

== system MMNNsExample1/b11(x1(t))*f(x1(t-tau1(t)))/x1(t)*b11(x1(t))/f=(|x+1|-|x-1|)//2 ==
  In1 : Inport
  Abs : Abs
  Abs1 : Abs
  Add : Sum  Inputs=+-
  Add1 : Sum
  Add2 : Sum  Inputs=+-
  Constant : Constant
  Constant1 : Constant
  Gain : Gain  Gain=0.5
  Out1 : Outport
  wires:
  Constant1/1 -> Add1/1
  In1/1 -> Add/1, Add1/2
  Add1/1 -> Abs/1
  Abs/1 -> Add2/1
  Constant/1 -> Add/2
  Add/1 -> Abs1/1
  Abs1/1 -> Add2/2
  Add2/1 -> Gain/1
  Gain/1 -> Out1/1

== system MMNNsExample1/b11(x1(t))*f(x1(t-tau1(t)))/x1(t)*b11(x1(t))/tau1(t)=0.5+0.5*cos(t) ==
  Add : Sum
  Clock : Clock
  Constant : Constant
  Gain : Gain
  Gain1 : Gain  Gain=0.5
  Sine Wave Function : Sin  TimeSource=Use external signal  Phase=0.5*pi  SampleTime=0
      settings: AttributesFormatString=%<Name>
  tau(t)=0.5+0.5*cos(t) : Outport
  wires:
  Sine Wave Function/1 -> Gain/1  "cos(t)"
  Constant/1 -> Add/2
  Clock/1 -> Sine Wave Function/1
  Add/1 -> Gain1/1
  Gain/1 -> Add/1
  Gain1/1 -> tau(t)=0.5+0.5*cos(t)/1

== system MMNNsExample1/b22(1)(x2(t))*f(x2(t-tau1(t)))/x2(t)*b22(x2(t))/f(x(t))=0.5*(|x+1|-|x-1|) ==
  In1 : Inport
  Abs : Abs
  Abs1 : Abs
  Add : Sum  Inputs=+-
  Add1 : Sum
  Add2 : Sum  Inputs=+-
  Constant : Constant
  Constant1 : Constant
  Gain : Gain  Gain=0.5
  Out1 : Outport
  wires:
  Constant1/1 -> Add1/1
  In1/1 -> Add/1, Add1/2
  Add1/1 -> Abs/1
  Abs/1 -> Add2/1
  Constant/1 -> Add/2
  Add/1 -> Abs1/1
  Abs1/1 -> Add2/2
  Add2/1 -> Gain/1
  Gain/1 -> Out1/1

== system MMNNsExample1/b22(1)(x2(t))*f(x2(t-tau1(t)))/x2(t)*b22(x2(t))/tau(t)=0.5+0.5*cos(t) ==
  Add : Sum
  Clock : Clock
  Constant : Constant
  Gain : Gain
  Gain1 : Gain  Gain=0.5
  Sine Wave Function : Sin  TimeSource=Use external signal  Phase=0.5*pi  SampleTime=0
      settings: AttributesFormatString=%<Name>
  Out1 : Outport
  wires:
  Add/1 -> Gain1/1
  Clock/1 -> Sine Wave Function/1
  Sine Wave Function/1 -> Gain/1  "cos(t)"
  Constant/1 -> Add/2
  Gain/1 -> Add/1
  Gain1/1 -> Out1/1  "tau(t)=0.5+0.5*cos(t)"

== system MMNNsExample1/b22(2)(x2(t))*f(x2(t-tau2(t)))/x2(t)*b22(x2(t))/f(x(t))=0.5*(|x+1|-|x-1|) ==
  In1 : Inport
  Abs : Abs
  Abs1 : Abs
  Add : Sum  Inputs=+-
  Add1 : Sum
  Add2 : Sum  Inputs=+-
  Constant : Constant
  Constant1 : Constant
  Gain : Gain  Gain=0.5
  Out1 : Outport
  wires:
  Constant1/1 -> Add1/1
  In1/1 -> Add/1, Add1/2
  Add1/1 -> Abs/1
  Abs/1 -> Add2/1
  Constant/1 -> Add/2
  Add/1 -> Abs1/1
  Abs1/1 -> Add2/2
  Add2/1 -> Gain/1
  Gain/1 -> Out1/1

== system MMNNsExample1/b22(2)(x2(t))*f(x2(t-tau2(t)))/x2(t)*b22(x2(t))/tau2(t)=0.5+0.5*sin(t) ==
  Add : Sum
  Clock : Clock
  Constant : Constant
  Gain : Gain
  Gain1 : Gain  Gain=0.5
  Sine Wave Function : Sin  TimeSource=Use external signal  SampleTime=0
      settings: AttributesFormatString=%<Name>
  Out1 : Outport
  wires:
  Add/1 -> Gain1/1
  Clock/1 -> Sine Wave Function/1
  Sine Wave Function/1 -> Gain/1  "sin(t)"
  Constant/1 -> Add/2
  Gain/1 -> Add/1
  Gain1/1 -> Out1/1  "tau(t)=0.5+0.5*sin(t)"

== system MMNNsExample1/c11(x1(t))*inst(f(x1(t)))/c11*inst(f1(x1(t)))/d(rou(t))=0.5cos(t) ==
  Clock : Clock
  Gain : Gain  Gain=0.5
  Sine Wave Function : Sin  TimeSource=Use external signal  Phase=0.5*pi  SampleTime=0
  Out1 : Outport
  wires:
  Sine Wave Function/1 -> Gain/1  "cos(t)"
  Gain/1 -> Out1/1  "rou(t)=d(0.5+0.5*sin(t))"
  Clock/1 -> Sine Wave Function/1

== system MMNNsExample1/c11(x1(t))*inst(f(x1(t)))/c11*inst(f1(x1(t)))/f(x1(t)) ==
  In1 : Inport
  Abs : Abs
  Abs1 : Abs
  Add : Sum  Inputs=+-
  Add1 : Sum
  Add2 : Sum  Inputs=+-
  Constant1 : Constant
  Gain : Gain  Gain=0.5
  Out1 : Outport
  wires:
  Constant1/1 -> Add/2, Add1/1
  In1/1 -> Add/1, Add1/2  "x1(t)"
  Add1/1 -> Abs/1
  Abs/1 -> Add2/1
  Add/1 -> Abs1/1
  Abs1/1 -> Add2/2
  Add2/1 -> Gain/1
  Gain/1 -> Out1/1

== system MMNNsExample1/c11(x1(t))*inst(f(x1(t)))/c11*inst(f1(x1(t)))/f1(x1(t)) ==
  In1 : Inport
  Abs : Abs
  Abs1 : Abs
  Add : Sum  Inputs=+-
  Add1 : Sum
  Add2 : Sum  Inputs=+-
  Constant : Constant
  Constant1 : Constant
  Gain : Gain  Gain=0.5
  Out1 : Outport
  wires:
  Gain/1 -> Out1/1
  Add2/1 -> Gain/1
  Abs1/1 -> Add2/2
  Add/1 -> Abs1/1
  Constant/1 -> Add/2
  Abs/1 -> Add2/1
  Add1/1 -> Abs/1
  In1/1 -> Add1/2, Add/1
  Constant1/1 -> Add1/1

== system MMNNsExample1/c11(x1(t))*inst(f(x1(t)))/c11*inst(f1(x1(t)))/rou(t)=0.5+0.5*sin(t) ==
  Add : Sum
  Clock : Clock
  Constant : Constant
  Gain : Gain
  Gain1 : Gain  Gain=0.5
  Sine Wave Function : Sin  TimeSource=Use external signal  SampleTime=0
  Out1 : Outport
  wires:
  Clock/1 -> Sine Wave Function/1
  Constant/1 -> Add/2
  Gain/1 -> Add/1
  Add/1 -> Gain1/1
  Sine Wave Function/1 -> Gain/1  "sin(t)"
  Gain1/1 -> Out1/1

== system MMNNsExample1/c12(x1(t))*x2(t)/Subsystem/d(t-(rou(t))) ==
  Add : Sum  Inputs=+-
  Clock : Clock
  Constant2 : Constant
  Gain : Gain  Gain=0.5
  Sine Wave Function : Sin  TimeSource=Use external signal  Phase=0.5*pi  SampleTime=0
      settings: AttributesFormatString=%<Name>
  Out1 : Outport
  wires:
  Clock/1 -> Sine Wave Function/1
  Constant2/1 -> Add/1
  Gain/1 -> Add/2
  Add/1 -> Out1/1
  Sine Wave Function/1 -> Gain/1  "cos(t)"

== system MMNNsExample1/c12(x1(t))*x2(t)/Subsystem/f(x(t)))=0.5*(|x+1|-|x-1|) ==
  In1 : Inport
      settings: AttributesFormatString=%<Name>
  Abs : Abs
      settings: AttributesFormatString=%<Name>
  Abs1 : Abs
  Add : Sum
  Add1 : Sum  Inputs=-+
  Add2 : Sum  Inputs=+-
  Constant : Constant
  Gain : Gain  Gain=0.5
  Out1 : Outport
      settings: AttributesFormatString=%<Name>
  wires:
  Gain/1 -> Out1/1
  Abs/1 -> Add2/1
  Add2/1 -> Gain/1
  Add1/1 -> Abs1/1
  In1/1 -> Add1/2, Add/1
  Abs1/1 -> Add2/2
  Constant/1 -> Add1/1, Add/2
  Add/1 -> Abs/1

== system MMNNsExample1/c12(x1(t))*x2(t)/Subsystem/rou(t)=0.5*(1+sin(t)) ==
  Add2 : Sum
  Clock1 : Clock
  Constant3 : Constant
  Gain1 : Gain  Gain=0.5
  Sine Wave Function1 : Sin  TimeSource=Use external signal  SampleTime=0
      settings: AttributesFormatString=%<Name>
  Out1 : Outport
  wires:
  Constant3/1 -> Add2/2
  Sine Wave Function1/1 -> Add2/1  "sin(t)"
  Gain1/1 -> Out1/1  "rou(t)=0.5*(1+sin(t))"
  Add2/1 -> Gain1/1
  Clock1/1 -> Sine Wave Function1/1

== system MMNNsExample1/c21(x2(t))*inst(f(x1(t)))/Subsystem/d(t-(rou(t))) ==
  Add : Sum  Inputs=+-
  Clock : Clock
  Constant2 : Constant
  Gain : Gain  Gain=0.5
  Sine Wave Function : Sin  TimeSource=Use external signal  Phase=0.5*pi  SampleTime=0
      settings: AttributesFormatString=%<Name>
  Out1 : Outport
  wires:
  Clock/1 -> Sine Wave Function/1
  Constant2/1 -> Add/1
  Gain/1 -> Add/2
  Add/1 -> Out1/1
  Sine Wave Function/1 -> Gain/1  "cos(t)"

== system MMNNsExample1/c21(x2(t))*inst(f(x1(t)))/Subsystem/f(x(t))=0.5*(|x+1|-|x-1|) ==
  In1 : Inport
      settings: AttributesFormatString=%<Name>
  Abs : Abs
      settings: AttributesFormatString=%<Name>
  Abs1 : Abs
  Add : Sum
  Add1 : Sum  Inputs=-+
  Add2 : Sum  Inputs=+-
  Constant : Constant
  Gain : Gain  Gain=0.5
  Out1 : Outport
      settings: AttributesFormatString=%<Name>
  wires:
  Gain/1 -> Out1/1
  Abs/1 -> Add2/1
  Add2/1 -> Gain/1
  Add1/1 -> Abs1/1
  In1/1 -> Add1/2, Add/1
  Abs1/1 -> Add2/2
  Constant/1 -> Add1/1, Add/2
  Add/1 -> Abs/1

== system MMNNsExample1/c21(x2(t))*inst(f(x1(t)))/Subsystem/rou(t)=0.5*(1+sin(t)) ==
  Add2 : Sum
  Clock1 : Clock
  Constant3 : Constant
  Gain1 : Gain  Gain=0.5
  Sine Wave Function1 : Sin  TimeSource=Use external signal  SampleTime=0
      settings: AttributesFormatString=%<Name>
  Out1 : Outport
  wires:
  Constant3/1 -> Add2/2
  Sine Wave Function1/1 -> Add2/1  "sin(t)"
  Gain1/1 -> Out1/1
  Add2/1 -> Gain1/1
  Clock1/1 -> Sine Wave Function1/1

== system MMNNsExample1/c22(x2(t))*inst(f(x2(t)))/c22*inst(f2(x2(t)))/d(rou(t)) ==
  Clock : Clock
  Gain : Gain  Gain=0.5
  Sine Wave Function : Sin  TimeSource=Use external signal  Phase=0.5*pi  SampleTime=0
  Out1 : Outport
  wires:
  Sine Wave Function/1 -> Gain/1  "cos(t)"
  Gain/1 -> Out1/1  "d(rou(t))=0.5*cos(t)"
  Clock/1 -> Sine Wave Function/1

== system MMNNsExample1/c22(x2(t))*inst(f(x2(t)))/c22*inst(f2(x2(t)))/f(x(t))=0.5*(|x+1|-|x-1|) ==
  In1 : Inport
  Abs : Abs
  Abs1 : Abs
  Add : Sum  Inputs=+-
  Add1 : Sum
  Add2 : Sum  Inputs=+-
  Constant1 : Constant
  Gain : Gain  Gain=0.5
  Out1 : Outport
  wires:
  Constant1/1 -> Add/2, Add1/1
  In1/1 -> Add/1, Add1/2  "x1(t)"
  Add1/1 -> Abs/1
  Abs/1 -> Add2/1
  Add/1 -> Abs1/1
  Abs1/1 -> Add2/2
  Add2/1 -> Gain/1
  Gain/1 -> Out1/1

== system MMNNsExample1/c22(x2(t))*inst(f(x2(t)))/c22*inst(f2(x2(t)))/f2(x2(t))=0.5*(|x+1|-|x-1|) ==
  In1 : Inport
  Abs : Abs
  Abs1 : Abs
  Add : Sum  Inputs=+-
  Add1 : Sum
  Add2 : Sum  Inputs=+-
  Constant : Constant
  Constant1 : Constant
  Gain : Gain  Gain=0.5
  Out1 : Outport
  wires:
  Gain/1 -> Out1/1
  Add2/1 -> Gain/1
  Abs1/1 -> Add2/2
  Add/1 -> Abs1/1
  Constant/1 -> Add/2
  Abs/1 -> Add2/1
  Add1/1 -> Abs/1
  In1/1 -> Add1/2, Add/1
  Constant1/1 -> Add1/1

== system MMNNsExample1/c22(x2(t))*inst(f(x2(t)))/c22*inst(f2(x2(t)))/rou(t)=0.5(1+sin(t)) ==
  Add : Sum
  Clock : Clock
  Constant : Constant
  Gain : Gain  Gain=0.5
  Sine Wave Function : Sin  TimeSource=Use external signal  SampleTime=0
  Out1 : Outport
  wires:
  Clock/1 -> Sine Wave Function/1
  Constant/1 -> Add/2
  Add/1 -> Gain/1
  Sine Wave Function/1 -> Add/1  "sin(t)"
  Gain/1 -> Out1/1
